simulink model "RosslerSim"  (R2021a)
settings: Solver=VariableStepAuto  StartTime=0.0  StopTime=200  RelTol=1e-3
libraries: simulink x1
settings Model: Creator=timmy  LastModifiedBy=timmy

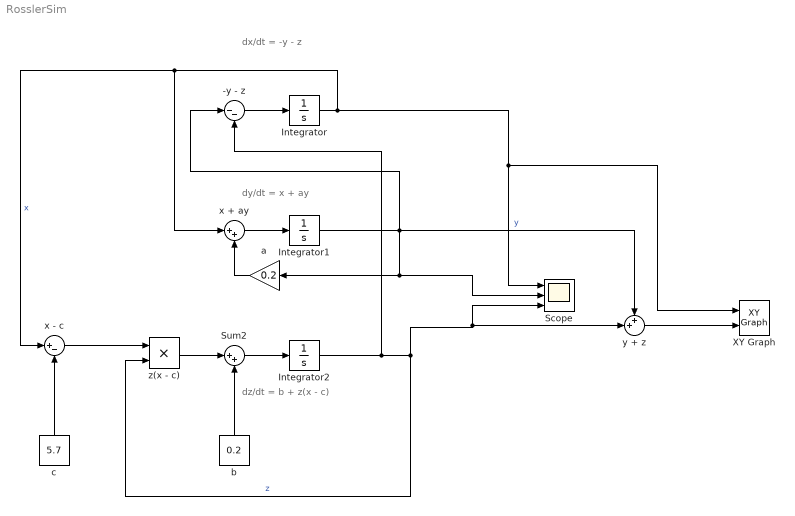
== system RosslerSim ==
  note: dx/dt = -y - z
  note: dy/dt = x + ay
  note: dz/dt = b + z(x - c)
  -y - z : Sum  Inputs=|--
  "Integrator " : Integrator
  Integrator1 : Integrator
  Integrator2 : Integrator
  Scope : Scope  NumInputPorts=3
  Sum2 : Sum  Inputs=|++
  XY Graph : simulink/Sinks/XY Graph  xmin=-10  xmax=15  ymin=-10  ymax=25  st=-1
  a : Gain  Gain=0.2
  b : Constant  Value=0.2
  c : Constant  Value=5.7
  x + ay : Sum  Inputs=|++
  x - c : Sum  Inputs=|+-
  y + z : Sum  Inputs=++|
  z(x - c) : Product
  wires:
  -y - z/1 -> "Integrator "/1
  x + ay/1 -> Integrator1/1
  Sum2/1 -> Integrator2/1
  z(x - c)/1 -> Sum2/1
  b/1 -> Sum2/2
  Integrator2/1 -> Scope/3, y + z/2, z(x - c)/2, -y - z/2  "z"
  c/1 -> x - c/2
  "Integrator "/1 -> XY Graph/1, Scope/1, x + ay/1, x - c/1  "x"
  Integrator1/1 -> y + z/1, a/1, Scope/2, -y - z/1  "y"
  a/1 -> x + ay/2
  x - c/1 -> z(x - c)/1
  y + z/1 -> XY Graph/2
